simulink model "Example"  (R2021b)
settings: Solver=ode14x  StartTime=0.0  StopTime=40  FixedStep=0.01  RelTol=1e-3
PreLoadFcn:
  | run('Example_init.m')
values from neighbouring files (symbols this model uses):
  A = BWB.lat.A    [Example_init.m]    (also in SMC1.m = BWB.A; SMCCanForm.m = Tr*A*Tr')
  B = BWB.lat.B    [Example_init.m]    (also in SMC1.m = BWB.B; SMCCanForm.m = Tr*B)
  C = eye(4)    [Example_init.m]
  Cc = [1 0 0 0 ... (first row only)    [Example_init.m]    (also in outfor.m = C*inv(Tc))
  D = zeros(4,8)    [Example_init.m]
libraries: SMC x1
settings Model: Creator=lev201  LastModifiedBy=Witali
settings SolverCC: AlgebraicLoopSolver=TrustRegion
settings DataIOCC: ReturnWorkspaceOutputs=off
settings DebuggingCC: SFMachineParentedDataDiag=warning  ArithmeticOperatorsInVariantConditions=warning
settings SFSimCC: SimUseLocalCustomCode=off  CustomCodeUndefinedFunction=UseInterfaceOnly
settings RTWCC: RTWUseLocalCustomCode=off

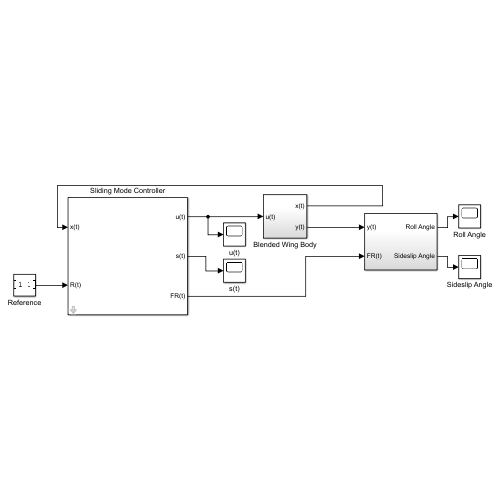
[thumbnail: Simulink's stored preview of the top-level diagram]
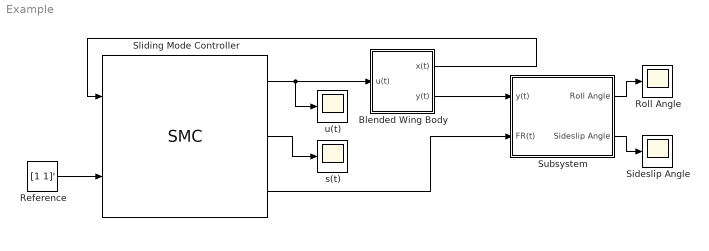
== system Example ==
  Blended Wing Body : Subsystem
  Reference : Constant  Value=[1 1]'
  Roll Angle : Scope
  Sideslip Angle : Scope
  Sliding Mode Controller : SMC/SMC  I=on  shs=on  adpt=off  showadpt=off  A=A  B=B  Cc=Cc  Q=Q  rho=15  C0=1  PC=1  K0=1  PK=1  delta=0.01  eps=0  Qi=Qi  Fil=on  Filter=F  FRt=on
      settings: SourceProductName=Sliding Mode Control Toolbox
  Subsystem : Subsystem
  s(t) : Scope
  u(t) : Scope
  wires:
  Reference/1 -> Sliding Mode Controller/2
  Blended Wing Body/1(x(t)) -> Sliding Mode Controller/1
  Sliding Mode Controller/1 -> u(t)/1, Blended Wing Body/1(u(t))
  Blended Wing Body/2(y(t)) -> Subsystem/1(y(t))
  Subsystem/1(Roll Angle) -> Roll Angle/1
  Subsystem/2(Sideslip Angle) -> Sideslip Angle/1
  Sliding Mode Controller/2 -> s(t)/1
  Sliding Mode Controller/3 -> Subsystem/2(FR(t))

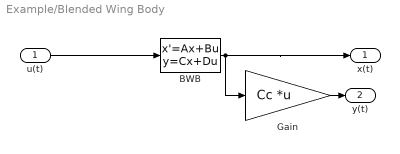
== system Example/Blended Wing Body ==
  u(t) : Inport
  BWB : StateSpace  A=A  B=B  C=C  D=D  InitialCondition=[0 0.1 0 0]
  Gain : Gain  Gain=Cc  Multiplication=Matrix(K*u) (u vector)
  x(t) : Outport  VectorParamsAs1DForOutWhenUnconnected=off
  y(t) : Outport  Port=2  VectorParamsAs1DForOutWhenUnconnected=off
  wires:
  u(t)/1 -> BWB/1
  BWB/1 -> Gain/1, x(t)/1
  Gain/1 -> y(t)/1

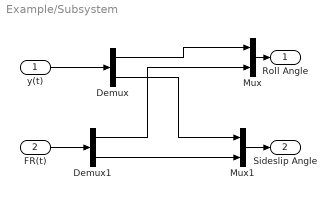
== system Example/Subsystem ==
  y(t) : Inport
  FR(t) : Inport  Port=2
  Demux : Demux  Outputs=2
  Demux1 : Demux  Outputs=2
  Mux : Mux  Inputs=2
  Mux1 : Mux  Inputs=2
  Roll Angle : Outport  VectorParamsAs1DForOutWhenUnconnected=off
  Sideslip Angle : Outport  Port=2  VectorParamsAs1DForOutWhenUnconnected=off
  wires:
  y(t)/1 -> Demux/1
  Demux/1 -> Mux/1
  Mux/1 -> Roll Angle/1
  Mux1/1 -> Sideslip Angle/1
  Demux/2 -> Mux1/1
  FR(t)/1 -> Demux1/1
  Demux1/1 -> Mux/2
  Demux1/2 -> Mux1/2
